simulink model "cpss51"  (R2023b)
settings: Solver=VariableStepAuto  StartTime=0.0  StopTime=10.0  RelTol=1e-3
libraries: simulink x11
settings Model: Creator=iceki  LastModifiedBy=iceki

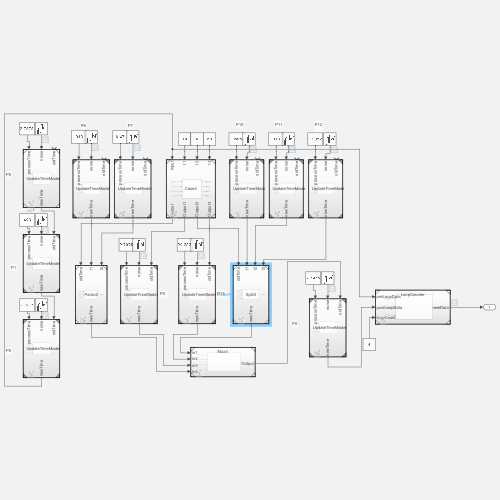
[thumbnail: Simulink's stored preview of the top-level diagram]
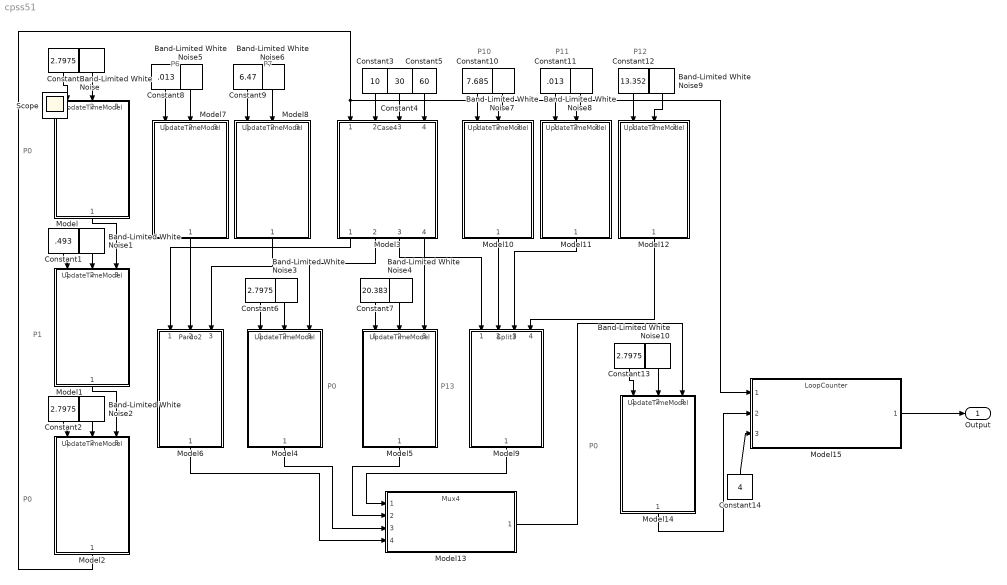
== system cpss51 ==
  note: P10
  note: P7
  note: P6
  note: P1
  note: P0
  note: P0
  note: P0
  note: P13
  note: P11
  note: P12
  note: P0
  Band-Limited White Noise{,1..10} (11 alike) : simulink/Sources/Band-Limited White Noise  Cov=[0.1]  Ts=0.1  seed=[23341]
  Constant{,2,6,13} (4 alike) : Constant  Value=2.7975
  Constant1 : Constant  Value=.493
  Constant10 : Constant  Value=7.685
  Constant11 : Constant  Value=.013
  Constant12 : Constant  Value=13.352
  Constant14 : Constant  Value=4
  Constant3 : Constant  Value=10
  Constant4 : Constant  Value=30
  Constant5 : Constant  Value=60
  Constant7 : Constant  Value=20.383
  Constant8 : Constant  Value=.013
  Constant9 : Constant  Value=6.47
  Model{,1..2,4..5,7..8,10..12,14} (11 alike) : ModelReference  ModelNameDialog=UpdateTimeModel.slx  SimulationMode=Normal  ModelReferenceVersion=3.0
  Model13 : ModelReference  ModelNameDialog=Mux4.slx  SimulationMode=Normal  ModelReferenceVersion=1.3
  Model15 : ModelReference  ModelNameDialog=LoopCounter.slx  SimulationMode=Normal  ModelReferenceVersion=1.1
  Model3 : ModelReference  ModelNameDialog=Case4.slx  SimulationMode=Normal  ModelReferenceVersion=1.6
  Model6 : ModelReference  ModelNameDialog=Pardo2.slx  SimulationMode=Normal  ModelReferenceVersion=1.9
  Model9 : ModelReference  ModelNameDialog=Split3.slx  SimulationMode=Normal  ModelReferenceVersion=1.6
  Output : Outport
  Scope : Scope
  wires:
  Constant/1 -> Model/1
  Band-Limited White Noise/1 -> Model/2
  Band-Limited White Noise1/1 -> Model1/2
  Constant1/1 -> Model1/1
  Model/1 -> Model1/3
  Band-Limited White Noise2/1 -> Model2/2
  Constant2/1 -> Model2/1
  Model1/1 -> Model2/3
  Model2/1 -> Model15/1, Model3/1
  Constant3/1 -> Model3/2
  Constant4/1 -> Model3/3
  Constant5/1 -> Model3/4
  Band-Limited White Noise3/1 -> Model4/2
  Constant6/1 -> Model4/1
  Model3/2 -> Model4/3
  Constant7/1 -> Model5/1
  Band-Limited White Noise4/1 -> Model5/2
  Model3/4 -> Model5/3
  Constant8/1 -> Model7/1
  Band-Limited White Noise5/1 -> Model7/2
  Band-Limited White Noise6/1 -> Model8/2
  Constant9/1 -> Model8/1
  Model7/1 -> Model6/2
  Model8/1 -> Model6/3
  Model3/1 -> Model6/1
  Model3/3 -> Model9/1
  ? -> ?
  Model10/1 -> Model9/2
  Model11/1 -> Model9/3
  Model12/1 -> Model9/4
  Constant10/1 -> Model10/1
  Band-Limited White Noise7/1 -> Model10/2
  Band-Limited White Noise8/1 -> Model11/2
  Constant11/1 -> Model11/1
  Band-Limited White Noise9/1 -> Model12/2
  Constant12/1 -> Model12/1
  Model9/1 -> Model13/1
  Model5/1 -> Model13/2
  Model4/1 -> Model13/3
  Model6/1 -> Model13/4
  Band-Limited White Noise10/1 -> Model14/2
  Constant13/1 -> Model14/1
  Model13/1 -> Model14/3
  Model14/1 -> Model15/2
  Constant14/1 -> Model15/3
  Model15/1 -> Output/1
